simulink model "ex1_simulink_design_and_sim"  (R2021b)
settings: Solver=VariableStepAuto  StartTime=0.0  StopTime=10.0  RelTol=1e-7
settings Model: Creator=steven  LastModifiedBy=steven

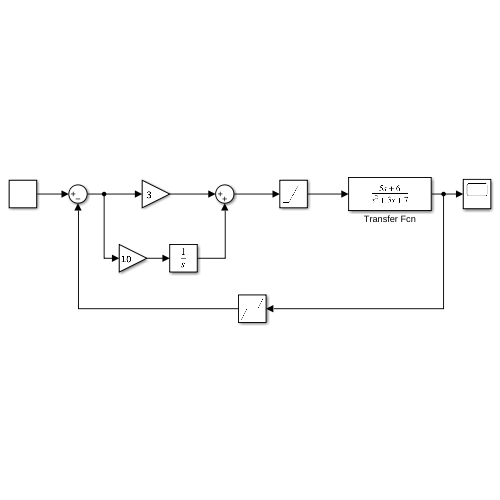
[thumbnail: Simulink's stored preview of the top-level diagram]
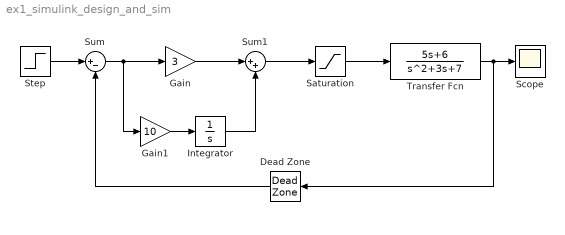
== system ex1_simulink_design_and_sim ==
  Dead Zone : DeadZone  LowerValue=-0.1  UpperValue=0.1  SaturateOnIntegerOverflow=on
  Gain : Gain  Gain=3
  Gain1 : Gain  Gain=10
  Integrator : Integrator
  Saturation : Saturate  UpperLimit=2  LowerLimit=-2
  Scope : Scope
  Step : Step  Time=0  SampleTime=0  ZeroCross=off
  Sum : Sum  Inputs=|+-
  Sum1 : Sum  Inputs=|++
  Transfer Fcn : TransferFcn  Numerator=[5 6]  Denominator=[1 3 7]
  wires:
  Step/1 -> Sum/1
  Saturation/1 -> Transfer Fcn/1
  Gain/1 -> Sum1/1
  Sum1/1 -> Saturation/1
  Transfer Fcn/1 -> Dead Zone/1, Scope/1
  Integrator/1 -> Sum1/2
  Gain1/1 -> Integrator/1
  Sum/1 -> Gain1/1, Gain/1
  Dead Zone/1 -> Sum/2
